simulink model "sailboat_simulation"  (R2018a)
settings: Solver=FixedStepDiscrete  StartTime=0.0  StopTime=1000  FixedStep=0.02  RelTol=1e-3  EnableMultiTasking=on
model workspace: external: MAT-File E:\实验课资料\matlab\ParInit.mat (data not in the file)
undefined symbols (not defined in the file): DiscIntNeverNeededParam
libraries: simulink x3
settings Model: NumberOfSteps=5  Creator=建云  LastModifiedBy=xiehq
settings DataIOCC: LimitDataPoints=on  SaveFormat=Array  SignalLoggingSaveFormat=ModelDataLogs
settings OptimizationCC: LifeSpan=inf
settings DebuggingCC: UnderspecifiedInitializationDetection=Classic  MergeDetectMultiDrivingBlocksExec=none  SolverPrmCheckMsg=warning  MultiTaskDSMMsg=warning  MultiTaskCondExecSysMsg=none  SFUnexpectedBacktrackingDiag=warning  SFNoUnconditionalDefaultTransitionDiag=warning  SFExecutionAtInitializationDiag=none
settings HardwareCC: ProdBitPerPointer=32  ProdBitPerSizeT=32  ProdBitPerPtrDiffT=32  ProdLargestAtomicFloat=None  ProdIntDivRoundTo=Undefined  ProdEndianess=Unspecified  ProdWordSize=32  ProdHWDeviceType=32-bit Generic
settings ModelReferenceCC: PropagateSignalLabelsOutOfModel=off
settings CodeAppCC: StateflowObjectComments=on
settings GRTTargetCC: TargetLangStandard=C89/C90 (ANSI)  GeneratePreprocessorConditionals=Disable all
settings ConfigComp: CovMetricSettings=dw  CovHtmlReporting=on  CovSaveCumulativeToWorkspaceVar=on  CovSaveSingleToWorkspaceVar=on  CovExternalEMLEnable=off

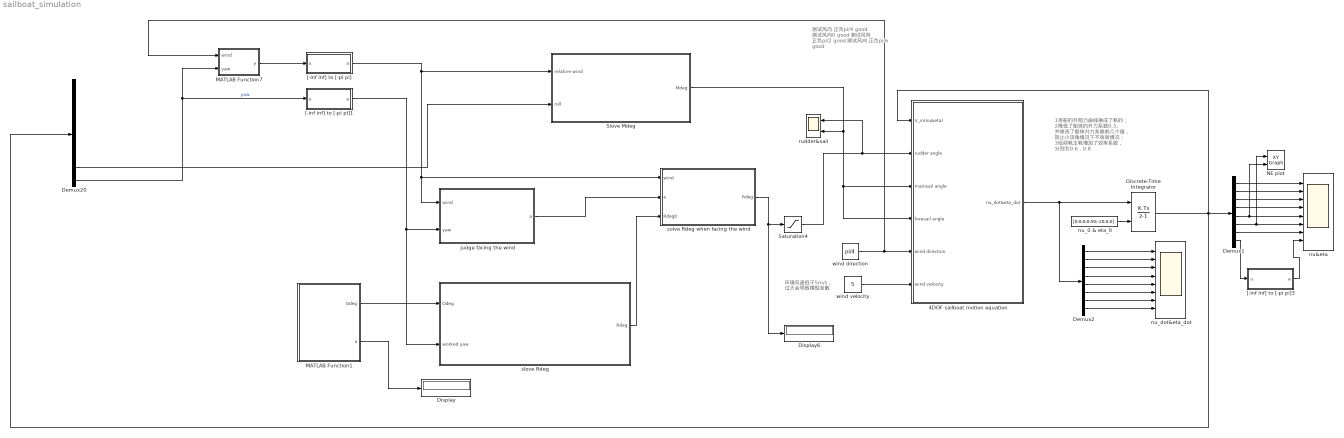
== system sailboat_simulation ==
  note: 环境风速低于5m/s，
      | 过大会导致模型发散
  note: 测试风向 正负pi/4 good
      | 测试风向0 good
      | 测试风向 正负pi/2 good
      | 测试风向 正负pi/6 good
  note: 1将舵的升阻力曲线换成了帆的；
      | 2降低了船体的升力系数0.3,
      | 并修改了船体升力系数前几个值，
      | 防止小攻角情况下不收敛情况；
      | 3给前帆主帆增加了效率系数，
      | 分别为0.6，0.8
  " Slove Mdeg" : Subsystem  TreatAsAtomicUnit=on
  4DOF sailboat motion equation : Subsystem
  Demux1 : Demux  Outputs=8
  Demux2 : Demux  Outputs=8
  Demux20 : Demux  Outputs=8
  Discrete-Time Integrator : DiscreteIntegrator  InitialConditionSource=external  SampleTime=-1  ICPrevOutput=DiscIntNeverNeededParam  ICPrevScaledInput=DiscIntNeverNeededParam
  Display : Display
  Display6 : Display
  MATLAB Function1 : MATLAB Function  TreatAsAtomicUnit=on
  MATLAB Function7 : MATLAB Function  TreatAsAtomicUnit=on
  NE plot : simulink/Sinks/XY Graph  xmin=-150  xmax=150  ymin=-150  ymax=150  st=-1
  Saturation4 : Saturate  UpperLimit=0.68  LowerLimit=-0.68
  "[-inf inf] to [-pi pi]" : MATLAB Function  TreatAsAtomicUnit=on
  "[-inf inf] to [-pi pi]1" : MATLAB Function  TreatAsAtomicUnit=on
  "[-inf inf] to [-pi pi]3" : MATLAB Function  TreatAsAtomicUnit=on
  "judge facing the wind " : MATLAB Function  TreatAsAtomicUnit=on
  nu&eta : Scope  NumInputPorts=8
  nu_0 & eta_0 : Constant  Value=[0;0;0;0;50;-20;0;0]
  nu_dot&eta_dot : Scope  NumInputPorts=8
  rudder&sail : Scope  NumInputPorts=2
  slove Rdeg : Subsystem  TreatAsAtomicUnit=on
  solve Rdeg when facing the wind : MATLAB Function  TreatAsAtomicUnit=on
  wind direction : Constant  Value=pi/4
  wind velocity : Constant  Value=5
  wires:
  nu_0 & eta_0/1 -> Discrete-Time Integrator/2
  Discrete-Time Integrator/1 -> Demux20/1, 4DOF sailboat motion equation/1(V_in(nu&eta)), Demux1/1
  Demux1/6 -> NE plot/1, nu&eta/6
  Demux1/4 -> nu&eta/4
  Demux1/5 -> NE plot/2, nu&eta/5
  Demux1/7 -> nu&eta/7
  Demux1/3 -> nu&eta/3
  Demux1/1 -> nu&eta/1
  Demux1/2 -> nu&eta/2
  Demux1/8 -> "[-inf inf] to [-pi pi]3"/1(u)
  " Slove Mdeg"/1(Mdeg) -> 4DOF sailboat motion equation/4(foresail angle), 4DOF sailboat motion equation/3(mainsail angle), rudder&sail/2
  wind velocity/1 -> 4DOF sailboat motion equation/6(wind velocity)
  4DOF sailboat motion equation/1(nu_dot&eta_dot) -> Demux2/1, Discrete-Time Integrator/1
  Demux2/6 -> nu_dot&eta_dot/6
  Demux2/4 -> nu_dot&eta_dot/4
  Demux2/5 -> nu_dot&eta_dot/5
  Demux2/7 -> nu_dot&eta_dot/7
  Demux2/3 -> nu_dot&eta_dot/3
  Demux2/1 -> nu_dot&eta_dot/1
  Demux2/2 -> nu_dot&eta_dot/2
  Demux2/8 -> nu_dot&eta_dot/8
  Saturation4/1 -> 4DOF sailboat motion equation/2(rudder angle), rudder&sail/1
  MATLAB Function1/1(Odeg) -> slove Rdeg/1(Odeg)
  wind direction/1 -> MATLAB Function7/1(wind), 4DOF sailboat motion equation/5(wind direction)
  "[-inf inf] to [-pi pi]1"/1(a) -> slove Rdeg/2(worked yaw), "judge facing the wind "/2(yaw)
  MATLAB Function7/1(y) -> "[-inf inf] to [-pi pi]"/1(u)
  Demux20/8 -> "[-inf inf] to [-pi pi]1"/1(u), MATLAB Function7/2(yaw)  "yaw"
  Demux20/7 -> " Slove Mdeg"/2(roll)
  solve Rdeg when facing the wind/1(Rdeg) -> Display6/1, Saturation4/1
  "judge facing the wind "/1(a) -> solve Rdeg when facing the wind/2(a)
  slove Rdeg/1(Rdeg) -> solve Rdeg when facing the wind/3(Rdeg0)
  "[-inf inf] to [-pi pi]"/1(a) -> solve Rdeg when facing the wind/1(wind), "judge facing the wind "/1(wind), " Slove Mdeg"/1(relative wind)
  "[-inf inf] to [-pi pi]3"/1(a) -> nu&eta/8
  MATLAB Function1/2(a) -> Display/1

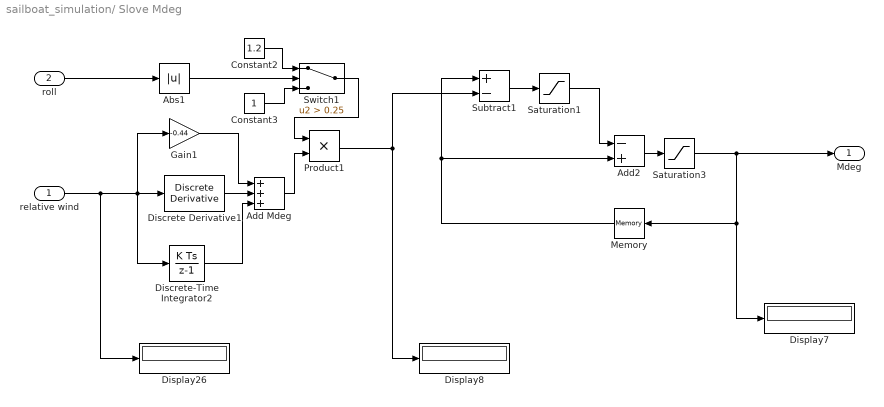
== system sailboat_simulation/ Slove Mdeg ==
  relative wind : Inport
  roll : Inport  Port=2
  Abs1 : Abs
  Add Mdeg : Sum  Inputs=+++
  Add2 : Sum  Inputs=-+
  Constant2 : Constant  Value=1.2
  Constant3 : Constant
  Discrete Derivative1 : simulink/Discrete/Discrete Derivative  gainval=-0.02  ICPrevScaledInput=0.0  InputProcessing=Inherited  OutMin=[]  OutMax=[]  OutDataType=fixdt(1, 16)  OutScaling=2^-10  DoSatur=off
  Discrete-Time Integrator2 : DiscreteIntegrator  gainval=0.00001  SampleTime=-1  ICPrevOutput=DiscIntNeverNeededParam  ICPrevScaledInput=DiscIntNeverNeededParam
  Display26 : Display
  Display7 : Display
  Display8 : Display
  Gain1 : Gain  Gain=-0.44
  Memory : Memory
  Product1 : Product
  Saturation1 : Saturate  UpperLimit=0.20  LowerLimit=-0.20
  Saturation3 : Saturate  UpperLimit=1.39  LowerLimit=-1.39
  Subtract1 : Sum  Inputs=+-
  Switch1 : Switch  Criteria=u2 > Threshold  Threshold=0.25
  Mdeg : Outport
  wires:
  Gain1/1 -> Add Mdeg/1
  Discrete Derivative1/1 -> Add Mdeg/2
  Discrete-Time Integrator2/1 -> Add Mdeg/3
  Subtract1/1 -> Saturation1/1
  Saturation1/1 -> Add2/1
  Memory/1 -> Subtract1/1, Add2/2
  Product1/1 -> Subtract1/2, Display8/1
  Constant3/1 -> Switch1/3
  Constant2/1 -> Switch1/1
  Add Mdeg/1 -> Product1/2
  Switch1/1 -> Product1/1
  Abs1/1 -> Switch1/2
  relative wind/1 -> Display26/1, Discrete-Time Integrator2/1, Gain1/1, Discrete Derivative1/1
  Saturation3/1 -> Memory/1, Display7/1, Mdeg/1
  roll/1 -> Abs1/1
  Add2/1 -> Saturation3/1

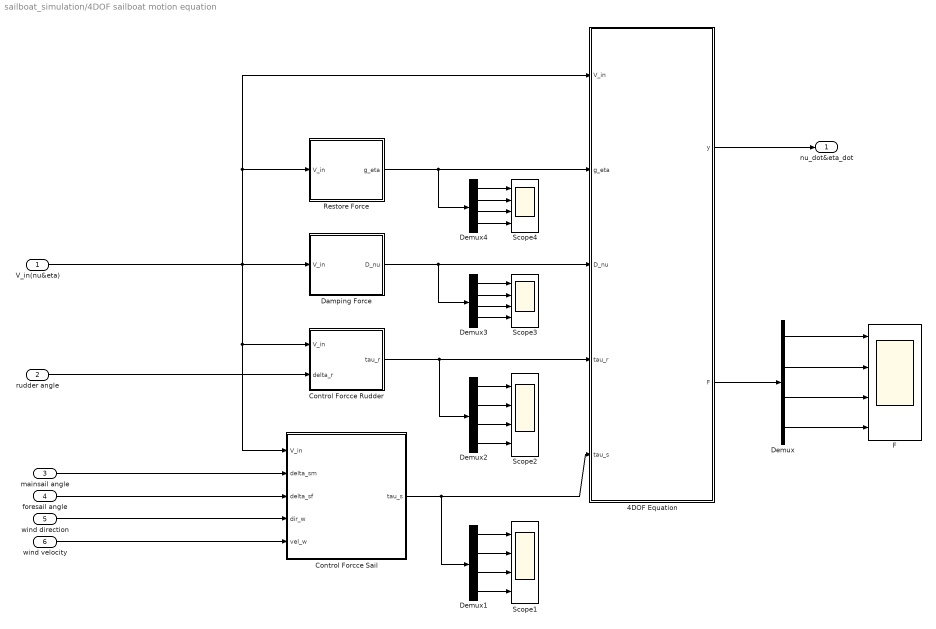
== system sailboat_simulation/4DOF sailboat motion equation ==
  V_in(nu&eta) : Inport
  rudder angle : Inport  Port=2
  mainsail angle : Inport  Port=3
  foresail angle : Inport  Port=4
  wind direction : Inport  Port=5
  wind velocity : Inport  Port=6
  4DOF Equation : MATLAB Function  TreatAsAtomicUnit=on
  Control Forcce Rudder : MATLAB Function  TreatAsAtomicUnit=on
  Control Forcce Sail : MATLAB Function  TreatAsAtomicUnit=on
  Damping Force : MATLAB Function  TreatAsAtomicUnit=on
  Demux{,1..4} (5 alike) : Demux
  F : Scope  NumInputPorts=4
  Restore Force : MATLAB Function  TreatAsAtomicUnit=on
  Scope{1..4} (4 alike) : Scope  NumInputPorts=4
  nu_dot&eta_dot : Outport
  wires:
  4DOF Equation/1(y) -> nu_dot&eta_dot/1
  V_in(nu&eta)/1 -> Damping Force/1(V_in), Control Forcce Sail/1(V_in), Control Forcce Rudder/1(V_in), Restore Force/1(V_in), 4DOF Equation/1(V_in)
  rudder angle/1 -> Control Forcce Rudder/2(delta_r)
  mainsail angle/1 -> Control Forcce Sail/2(delta_sm)
  foresail angle/1 -> Control Forcce Sail/3(delta_sf)
  wind velocity/1 -> Control Forcce Sail/5(vel_w)
  wind direction/1 -> Control Forcce Sail/4(dir_w)
  4DOF Equation/2(F) -> Demux/1
  Demux/1 -> F/1
  Demux/2 -> F/2
  Demux/4 -> F/4
  Demux/3 -> F/3
  Control Forcce Sail/1(tau_s) -> Demux1/1, 4DOF Equation/5(tau_s)
  Demux1/1 -> Scope1/1
  Demux1/2 -> Scope1/2
  Demux1/4 -> Scope1/4
  Demux1/3 -> Scope1/3
  Control Forcce Rudder/1(tau_r) -> Demux2/1, 4DOF Equation/4(tau_r)
  Demux2/1 -> Scope2/1
  Demux2/2 -> Scope2/2
  Demux2/4 -> Scope2/4
  Demux2/3 -> Scope2/3
  Damping Force/1(D_nu) -> Demux3/1, 4DOF Equation/3(D_nu)
  Demux3/1 -> Scope3/1
  Demux3/2 -> Scope3/2
  Demux3/4 -> Scope3/4
  Demux3/3 -> Scope3/3
  Restore Force/1(g_eta) -> Demux4/1, 4DOF Equation/2(g_eta)
  Demux4/1 -> Scope4/1
  Demux4/2 -> Scope4/2
  Demux4/4 -> Scope4/4
  Demux4/3 -> Scope4/3

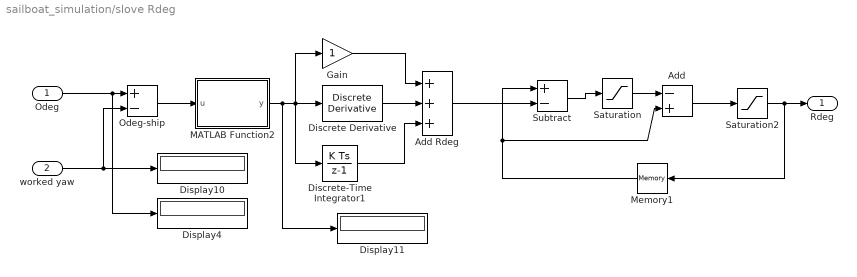
== system sailboat_simulation/slove Rdeg ==
  Odeg : Inport
  worked yaw : Inport  Port=2
  Add : Sum  Inputs=-+
  Add Rdeg : Sum  Inputs=+++
  Discrete Derivative : simulink/Discrete/Discrete Derivative  gainval=0.05  ICPrevScaledInput=0.0  InputProcessing=Inherited  OutMin=[]  OutMax=[]  OutDataType=fixdt(1, 16)  OutScaling=2^-10  DoSatur=off
  Discrete-Time Integrator1 : DiscreteIntegrator  gainval=0.001  SampleTime=-1  ICPrevOutput=DiscIntNeverNeededParam  ICPrevScaledInput=DiscIntNeverNeededParam
  Display10 : Display
  Display11 : Display
  Display4 : Display
  Gain : Gain
  MATLAB Function2 : MATLAB Function  TreatAsAtomicUnit=on
  Memory1 : Memory
  Odeg-ship : Sum  Inputs=+-
  Saturation : Saturate  UpperLimit=0.175  LowerLimit=-0.175
  Saturation2 : Saturate  UpperLimit=0.68  LowerLimit=-0.68
  Subtract : Sum  Inputs=+-
  Rdeg : Outport
  wires:
  Odeg/1 -> Display4/1, Odeg-ship/1
  Gain/1 -> Add Rdeg/1
  Discrete Derivative/1 -> Add Rdeg/2
  Subtract/1 -> Saturation/1
  Saturation/1 -> Add/1
  Add Rdeg/1 -> Subtract/2
  Memory1/1 -> Subtract/1, Add/2
  Discrete-Time Integrator1/1 -> Add Rdeg/3
  Odeg-ship/1 -> MATLAB Function2/1(u)
  worked yaw/1 -> Odeg-ship/2, Display10/1
  Add/1 -> Saturation2/1
  MATLAB Function2/1(y) -> Display11/1, Discrete Derivative/1, Gain/1, Discrete-Time Integrator1/1
  Saturation2/1 -> Memory1/1, Rdeg/1

== matlab function sailboat_simulation/4DOF sailboat motion equation/Restore Force ==
  data: par parameter; V_in input; g_eta output
function g_eta = fcn(par,V_in)
phi = V_in(7);
g_eta = [         0
                  0
         par.m*par.g*par.GMt*sin(phi)*cos(phi)
                  0 ];
end

== matlab function sailboat_simulation/4DOF sailboat motion equation/4DOF Equation ==
  data: par parameter; V_in input; y output; g_eta input; D_nu input; tau_r input; tau_s input; F output
function [y,F] = fcn(par,V_in,g_eta,D_nu,tau_r,tau_s)
%#codegen
nu = V_in(1:4);
u = nu(1);
v = nu(2);
p = nu(3);
r = nu(4);
eta = V_in(5:8);
phi = eta(3); % heel angle
psi = eta(4); % yaw angle

%% Rigid body Inertia Matrix & Coriolis-centripetal Matrix
M_RB = [  par.m           0            0                0
            0           par.m     -par.m*par.z_g  par.m*par.x_g
            0        -par.m*par.z_g   par.Ix         -par.Ixz
            0         par.m*par.x_g  -par.Ixz         par.Iz  ];
        
C_RB = [    0             0        par.m*par.z_g*r     -par.m*(par.x_g*r+v)
            0             0               0             par.m*u
    -par.m*par.z_g*r      0               0                0
   par.m*(par.x_g*r+v)  -par.m*u           0                0  ];

%% Added mass Inertia Matrix & Coriolis-centripetal Matrix
M_A = [  par.a11       0           0          0
            0      par.a22      par.a24    par.a26
            0      par.a24      par.a44    par.a46
            0      par.a26      par.a46    par.a66  ];
C_A = [   0                          0          0   -(par.a22*v+par.a24*p+par.a26*r)
          0                          0          0             par.a11*u
          0                          0          0                0
   par.a22*v+par.a24*p+par.a26*r -par.a11*u     0                0  ];

%%
M = M_RB + M_A;
C = C_RB + C_A;
% rank = rank(M)

J = [ cos(psi)  -sin(psi)*cos(phi)   0     0
      sin(psi)   cos(psi)*cos(phi)   0     0
         0               0           1     0
         0               0           0  cos(phi) ];   
     
F = -g_eta - D_nu + tau_r + tau_s;
     
nu_dot = M\(-C*nu+F);
% nu_dot = -M\(C_RB*nu+C_A*nu)-M\D_nu-M\g_eta+M\(tau_r+tau_s);
eta_dot = J*nu;

y = [nu_dot;eta_dot];

== matlab function sailboat_simulation/4DOF sailboat motion equation/Damping Force ==
  data: par parameter; V_in input; D_nu output
function D_nu= fcn(par,V_in)

nu = V_in(1:4);
phi_dot = nu(3);
psi_dot = nu(4)*cos(V_in(7));
%% translation damping

[Dk_nu,alpha_k] = Damping(nu,par.rou,par.Ak,par.x_k,par.y_k,par.z_k,'keel');
[Dh_nu,alpha_h] = Damping(nu,par.rou,par.Ah,par.x_h,par.y_h,par.z_h,'hull');
%% rotation damping

Dhk_eta = [       0
                  0
      par.k1*phi_dot*abs(phi_dot)
   par.k2*psi_dot*abs(psi_dot)*cos(V_in(7))  ];
%%
D_nu = Dk_nu + Dh_nu + Dhk_eta;

end

function [D_nu, alpha] = Damping(nu,rou,A,x,y,z,name)
u = nu(1);
v = nu(2);
p = nu(3);
r = nu(4);
v_au = -u + r*y;
v_av = -v - r*x + p*z;
alpha = atan2(-v_av,-v_au);
V2 = v_au^2 + v_av^2;
if strcmp(name, 'keel')
    [Cl,Cd] = keelcoef(alpha);
elseif strcmp(name,'hull')
    [Cl,Cd] = hullcoef(alpha);
end

k1 = 0.8; k2 = 1;
L = k1*0.5*rou*A*V2*Cl;
D = k2*0.5*rou*A*V2*Cd;
tmp1 = -L*sin(alpha)+D*cos(alpha);
tmp2 =  L*cos(alpha)+D*sin(alpha);
D_nu = [ tmp1
         tmp2
        -tmp2*z
         tmp2*x ];

end

function [Clk,Cdk] = keelcoef(attack)
% generate a lookup table for the lift/drag coefficients for the keel
% and compute Clk/Cdk from the lookup table using interpolation.

% lookup table
xdata = linspace(0,pi/2,37); % every 2.5 degrees
% lift curve
yldata = 0.8*[0, 0.2013, 0.4489, 0.7977, 1.003, 0.7512, 0.5264, 0.5447, 0.578,...
    0.6124, 0.6461, 0.6782, 0.7037, 0.7246, 0.7381, 0.7466, 0.7467, 0.7424,...
    0.7317, 0.7128, 0.6872, 0.656, 0.6206, 0.5822, 0.542, 0.5014, 0.4616,...
    0.4239, 0.387, 0.3486, 0.309, 0.2682, 0.2262, 0.183, 0.1389, 0.0937, 0.0476];
% drag curve
yddata = [0.0049, 0.0053, 0.0095, 0.0153, 0.0259, 0.1171, 0.1544, 0.1834,...
    0.2105, 0.2401, 0.27, 0.2998, 0.3313, 0.3617, 0.392, 0.4214, 0.4478,...
    0.4734, 0.5071, 0.5454, 0.5881, 0.635, 0.6861, 0.7413, 0.8004, 0.8633,...
    0.9298, 1.0, 1.077, 1.165, 1.263, 1.369, 1.483, 1.604, 1.731, 1.863, 2.0];

if attack>=0 && attack<=pi/2
    xp = attack;
    Clk = interp1(xdata,yldata,xp);
    Cdk = interp1(xdata,yddata,xp);
elseif attack>pi/2 && attack<=pi
    xp = pi-attack;
    Clk = -interp1(xdata,yldata,xp);
    Cdk = interp1(xdata,yddata,xp);
elseif attack>=-pi/2 && attack<0
    xp = -attack;
    Clk = -interp1(xdata,yldata,xp);
    Cdk = interp1(xdata,yddata,xp);
else
    xp = attack+pi;
    Clk = interp1(xdata,yldata,xp);
    Cdk = interp1(xdata,yddata,xp);
end
end

function [Clh,Cdh] = hullcoef(attack)
% generate a lookup table for the lift/drag coefficients for the hull
% and compute Clh/Cdh from the lookup table using interpolation.

% lookup table
xdata = linspace(0,pi/2,37); % every 2.5 degrees
% lift curve
yldata = 0.3*[0, 0.1541, 0.273, 0.544, 0.7884, 0.929, 1.043, 0.8797, 0.4805,...
    0.5259, 0.5735, 0.6195, 0.66, 0.6923, 0.7183, 0.7345, 0.7445, 0.745,...
    0.7383, 0.7271, 0.7125, 0.6945, 0.673, 0.6481, 0.6196, 0.5877, 0.5522,...
    0.5132, 0.4707, 0.4246, 0.3748, 0.3215, 0.2645, 0.2039, 0.1396, 0.0717, 0];
% drag curve
yddata = [0.0055, 0.0057, 0.0075, 0.0126, 0.0184, 0.0281, 0.0487, 0.1113,...
    0.1904, 0.2225, 0.2566, 0.2897, 0.3251, 0.3612, 0.3971, 0.4307, 0.465,...
    0.4935, 0.5206, 0.5583, 0.6006, 0.6478, 0.6999, 0.757, 0.8192, 0.8866,...
    0.9593, 1.037, 1.121, 1.21, 1.305, 1.406, 1.513, 1.625, 1.744, 1.869, 2.0];

if attack>=0 && attack<=pi/2
    xp = attack;
    Clh = interp1(xdata,yldata,xp);
    Cdh = interp1(xdata,yddata,xp);
elseif attack>pi/2 && attack<=pi
    xp = pi-attack;
    Clh = -interp1(xdata,yldata,xp);
    Cdh = interp1(xdata,yddata,xp);
elseif attack>=-pi/2 && attack<0
    xp = -attack;
    Clh = -interp1(xdata,yldata,xp);
    Cdh = interp1(xdata,yddata,xp);
else
    xp = attack+pi;
    Clh = interp1(xdata,yldata,xp);
    Cdh = interp1(xdata,yddata,xp);
end
end

== matlab function sailboat_simulation/4DOF sailboat motion equation/Control Forcce Rudder ==
  data: par parameter; V_in input; tau_r output; delta_r input
function tau_r= fcn(par,V_in,delta_r)

nu = V_in(1:4);
[beta,alpha,tau_r] = ControlForce(nu,par.rou,par.Ar,par.x_r,par.y_r,par.z_r,delta_r);

end

function [beta,alpha,tau] = ControlForce(nu,rou,A,x,y,z,delta)
u = nu(1);
v = nu(2);
p = nu(3);
r = nu(4);
v_au = -u + r*y;
v_av = -v - r*x + p*z;
beta = atan2(-v_av,-v_au);
tmp = delta + beta;
while abs(tmp)>pi
    if tmp>0
        tmp = tmp-2*pi;
    else
        tmp = tmp+2*pi;
    end
end
alpha = tmp;

V2 = v_au^2 + v_av^2;

[Cl,Cd] = ruddercoef(alpha);

k1 = 0.8; k2 = 0.8; %rudder effective coefficient
L = k1*0.5*rou*A*V2*Cl;
D = k2*0.5*rou*A*V2*Cd;
tmp1 = L*sin(alpha)-D*cos(alpha);
tmp2 = -L*cos(alpha)-D*sin(alpha);
tmp3 = tmp1*cos(delta)+tmp2*sin(delta);
tmp4 = -tmp1*sin(delta)+tmp2*cos(delta);
tau = [  tmp3
         tmp4
        -tmp4*z
         tmp4*x ];

end

function [Clr,Cdr] = ruddercoef(attack)
% generate a lookup table for the lift/drag coefficients for the rudder
% and compute Clr/Cdr from the lookup table using interpolation.

% lookup table
xdata = linspace(0,pi/2,37); % every 2.5 degrees
% lift curve
yldata = [0, 0.3212, 0.683, 0.8553, 0.9999, 1.095, 0.652, 0.6738, 0.7474,...
    0.8103, 0.8848, 0.9566, 1.024, 1.085, 1.14, 1.186, 1.222, 1.248, 1.018,...
    0.7698, 0.7468, 0.7174, 0.6837, 0.6453, 0.6056, 0.5646, 0.5223, 0.4784,...
    0.4329, 0.3858, 0.3368, 0.286, 0.2331, 0.1782, 0.1211, 0.0617, 0];
% drag curve
yddata = [ 0.0072, 0.009, 0.012, 0.0161, 0.0224, 0.0324, 0.1509, 0.1952,...
    0.2271, 0.2624, 0.2917, 0.3198, 0.3469, 0.3721, 0.3962, 0.418, 0.4338,...
    0.4466, 0.5092, 0.576, 0.5956, 0.6071, 0.6147, 0.6325, 0.663, 0.7062,...
    0.7621, 0.8305, 0.9114, 1.005, 1.11, 1.229, 1.359, 1.501, 1.655, 1.822, 2.0];

if attack>=0 && attack<=pi/2
    xp = attack;
    Clr = interp1(xdata,yldata,xp);
    Cdr = interp1(xdata,yddata,xp);
elseif attack>pi/2 && attack<=pi
    xp = pi-attack;
    Clr = -interp1(xdata,yldata,xp);
    Cdr = interp1(xdata,yddata,xp);
elseif attack>=-pi/2 && attack<0
    xp = -attack;
    Clr = -interp1(xdata,yldata,xp);
    Cdr = interp1(xdata,yddata,xp);
else
    xp = attack+pi;
    Clr = interp1(xdata,yldata,xp);
    Cdr = interp1(xdata,yddata,xp);
end
end

== matlab function sailboat_simulation/4DOF sailboat motion equation/Control Forcce Sail ==
  data: par parameter; V_in input; tau_s output; delta_sm input; delta_sf input; dir_w input; vel_w input
function tau_s= fcn(par,V_in,delta_sm,delta_sf,dir_w,vel_w)

nu = V_in(1:4);
eta = V_in(5:8);
phi = eta(3);
psi = eta(4);
J1 = [    cos(psi)         sin(psi)
    -cos(phi)*sin(psi)  cos(phi)*cos(psi) ];
v_twn = [vel_w*cos(dir_w);vel_w*sin(dir_w)];
v_twb = J1*v_twn;

x_sm = par.pm1-par.pm2*cos(delta_sm);
y_sm = par.pm2*sin(delta_sm);
z_sm = par.z_sm;

x_sf = par.pf1-par.pf2*cos(delta_sf);
y_sf = par.pf2*sin(delta_sf);
z_sf = par.z_sf;

k1 = 0.8; k2 = 0.6; % mail & fore sail effective coeff
tau_sm = k1*ControlForce(nu,par.rou1,par.Asm,x_sm,y_sm,z_sm,delta_sm,v_twb);
tau_sf = k2*ControlForce(nu,par.rou1,par.Asf,x_sf,y_sf,z_sf,delta_sf,v_twb);
tau_s = tau_sm + tau_sf;

end

function [tau] = ControlForce(nu,rou,A,x,y,z,delta,v_tw)
u = nu(1);
v = nu(2);
p = nu(3);
r = nu(4);
v_au = u - r*y;
v_av = v + r*x - p*z;
v_as = [v_au;v_av];
v_aw = v_tw - v_as;
beta = atan2(-v_aw(2),-v_aw(1));
tmp = delta + beta;
while abs(tmp)>pi
    if tmp>0
        tmp = tmp-2*pi;
    else
        tmp = tmp+2*pi;
    end
end
alpha = tmp;
% if tmp>=-pi && tmp<=pi
%     alpha = tmp;
% elseif tmp>pi
%     alpha = tmp-2*pi;
% else 
%     alpha = tmp+2*pi;
% end
V2 = v_aw(1)^2 + v_aw(2)^2;

[Cl,Cd] = sailcoef(alpha);

L = 0.5*rou*A*V2*Cl;
D = 0.5*rou*A*V2*Cd;
tmp1 = L*sin(alpha)-D*cos(alpha);
tmp2 = -L*cos(alpha)-D*sin(alpha);
tmp3 = tmp1*cos(delta)+tmp2*sin(delta);
tmp4 = -tmp1*sin(delta)+tmp2*cos(delta);
tau = [  tmp3
         tmp4
        -tmp4*z
         tmp4*x ];

end

function [Cls,Cds] = sailcoef(attack)
% generate a lookup table for the lift/drag coefficients for the sail
% and compute Cls/Cds from the lookup table using interpolation.

% lookup table
xdata = linspace(0,pi/2,37); % every 2.5 degrees
% lift curve
yldata = [0, 0.2212, 0.583, 0.8553, 0.9999, 1.095, 0.652, 0.6738, 0.7474,...
    0.8103, 0.8848, 0.9566, 1.024, 1.085, 1.14, 1.186, 1.222, 1.248, 1.018,...
    0.7698, 0.7468, 0.7174, 0.6837, 0.6453, 0.6056, 0.5646, 0.5223, 0.4784,...
    0.4329, 0.3858, 0.3368, 0.286, 0.2331, 0.1782, 0.1211, 0.0617, 0];
% drag curve
yddata = [ 0.0072, 0.009, 0.012, 0.0161, 0.0224, 0.0324, 0.1509, 0.1952,...
    0.2271, 0.2624, 0.2917, 0.3198, 0.3469, 0.3721, 0.3962, 0.418, 0.4338,...
    0.4466, 0.5092, 0.576, 0.5956, 0.6071, 0.6147, 0.6325, 0.663, 0.7062,...
    0.7621, 0.8305, 0.9114, 1.005, 1.11, 1.229, 1.359, 1.501, 1.655, 1.822, 2.0];

if attack>=0 && attack<=pi/2
    xp = attack;
    Cls = interp1(xdata,yldata,xp);
    Cds = interp1(xdata,yddata,xp);
elseif attack>pi/2 && attack<=pi
    xp = pi-attack;
    Cls = -interp1(xdata,yldata,xp);
    Cds = interp1(xdata,yddata,xp);
elseif attack>=-pi/2 && attack<0
    xp = -attack;
    Cls = -interp1(xdata,yldata,xp);
    Cds = interp1(xdata,yddata,xp);
else
    xp = attack+pi;
    Cls = interp1(xdata,yldata,xp);
    Cds = interp1(xdata,yddata,xp);
end
end

== matlab function sailboat_simulation/[-inf inf] to [-pi pi] ==
  data: a output; u input
function a  = fcn(u)
%#chushihua
while abs(u)>pi
    if u>pi
        u = u-2*pi;
    elseif u<-pi
        u = u+2*pi;
    end
end       
a = u;

== matlab function sailboat_simulation/MATLAB Function1 ==
  data: Odeg output; a output
function [Odeg,a] = fcn
%#codegen
time=0.02;
persistent k
if isempty(k)
    k = 0;
elseif k>=4000
    k=0;
else
    k = k+1;
end

if k<=40/time
    Odeg=0;
else 
    Odeg=pi;
end
a=k;

== matlab function sailboat_simulation/[-inf inf] to [-pi pi]1 ==
  data: a output; u input
function a  = fcn(u)
%#chushihua
while abs(u)>pi
    if u>pi
        u = u-2*pi;
    elseif u<-pi
        u = u+2*pi;
    end
end       
a = u;

== matlab function sailboat_simulation/[-inf inf] to [-pi pi]3 ==
  data: a output; u input
function a  = fcn(u)
%#chushihua
while abs(u)>pi
    if u>pi
        u = u-2*pi;
    elseif u<-pi
        u = u+2*pi;
    end
end       
a = u;

== matlab function sailboat_simulation/MATLAB Function7 ==
  data: wind input; y output; yaw input
function y = fcn(wind,yaw)
%#codegen
y=wind-yaw-pi;

== matlab function sailboat_simulation/solve Rdeg when facing the wind ==
  data: wind input; a input; Rdeg output; Rdeg0 input
function Rdeg  = fcn(wind,a,Rdeg0)
%#chushihua
persistent k;
persistent time;
persistent pdtime;
persistent Rdegtime;
persistent Rdeg1;
if isempty(k)
    k=1;
end
if isempty(time)
    time=1;
end
if isempty(pdtime)
    pdtime=0;
end
if isempty(Rdegtime)
    Rdegtime=0;
end
if isempty(Rdeg1)
    Rdeg1=0;
end
k=k+1;

%% panduan
if wind>0
    i=-1;
else
    i=1;
end
if a==1
    time=k;
    Rdegtime=i*0.1;
    pdtime=1;
end

if k>=time+200
    pdtime=0;
elseif k>=time+50
    pdtime=2;
end

if pdtime==1
    Rdeg=Rdegtime;
elseif pdtime==2
    Rdeg=0;
else
    Rdeg=Rdeg0;
end
x=pdtime;
deg=Rdeg1;

== matlab function sailboat_simulation/judge facing the wind  ==
  data: a output; wind input; yaw input
function a  = fcn(wind,yaw)
%#chushihua
persistent yaw1;
persistent yaw2;
persistent yaw3;
persistent yaw4;
persistent yaw5;
persistent yaw6;
persistent yaw7;
persistent yaw8;
persistent yaw9;
persistent yaw10;
persistent yaw11;
persistent yaw12;
persistent yaw13;
persistent yaw14;
persistent yaw15;
if isempty(yaw1)
    yaw1=0;
end
if isempty(yaw2)
    yaw2=0;
end
if isempty(yaw3)
    yaw3=0;
end
if isempty(yaw4)
    yaw4=0;
end
if isempty(yaw5)
    yaw5=0;
end
if isempty(yaw6)
    yaw6=0;
end
if isempty(yaw7)
    yaw7=0;
end
if isempty(yaw8)
    yaw8=0;
end
if isempty(yaw9)
    yaw9=0;
end
if isempty(yaw10)
    yaw10=0;
end
if isempty(yaw11)
    yaw11=0;
end
if isempty(yaw12)
    yaw12=0;
end
if isempty(yaw13)
    yaw13=0;
end
if isempty(yaw14)
    yaw14=0;
end
if isempty(yaw15)
    yaw15=0;
end

yaw15=yaw14;
yaw14=yaw13;
yaw13=yaw12;
yaw12=yaw11;
yaw11=yaw10;
yaw10=yaw9;
yaw9=yaw8;
yaw8=yaw7;
yaw7=yaw6;
yaw6=yaw5;
yaw5=yaw4;
yaw4=yaw3;
yaw3=yaw2;
yaw2=yaw1;
yaw1=yaw;

if abs(yaw1-yaw15)<0.05&&abs(wind)<0.65
    a=1;
else
    a=0;
end

== matlab function sailboat_simulation/slove Rdeg/MATLAB Function2 ==
  data: u input; y output
function y = fcn(u)
%#codegen
if u>pi
    y = u-2*pi;
elseif u<-pi
    y = u+2*pi;
else
    y=u;
end
